simulink model "nxtmouse"  (Simulink 6.4)
settings: Solver=ode4  StartTime=0.0  StopTime=inf  FixedStep=Ts  RelTol=1e-3
PreLoadFcn:
  | param;
values from neighbouring files (symbols this model uses):
  CAMERA_POS = [100 100]    [param.m]
  Cm = 9.00e-6    (= 9e-06)    [param.m]
  Cw = 9.00e-4    (= 0.0009)    [param.m]
  Dx = 1e-3    (= 0.001)    [param.m]
  Dzz = 1e-6    (= 1e-06)    [param.m]
  e = -0.2    [param.m]
  J = M*(W/2)^2    (= 0.004096)    [param.m]
  Jm = 0.5e-7    (= 5e-08)    [param.m]
  Jw = 20.0e-7    (= 2e-06)    [param.m]
  Kb = 0.022    [param.m]
  Kt = 0.022    [param.m]
  LENGTH = 20    [param.m]
  LENGTH2 = 16    [param.m]
  Lm = 1.4e-3    (= 0.0014)    [param.m]
  M = 0.64    [param.m]
  n = 24    [param.m]
  Rm = 1.0    (= 1)    [param.m]
  Rw = 0.056/2    (= 0.028)    [param.m]
  START_POS = [22 15]    [param.m]
  TRACK_MAP = double(imread('track.bmp'))    [param.m]
  Ts = 0.0001    [param.m]
  W = 0.16    [param.m]
  WALL_MAP = ~(TRACK_MAP - WALL)    [param.m]
  WIDTH = 16    [param.m]
  WIDTH1 = 12    [param.m]
undefined symbols (not defined in the file or in its folder): clearNXTSignalObjects, DiscIntNeverNeededParam
libraries: simulink x13, vrlib x1, ecrobot_nxt_lib x1
(part 1 of 3)
settings Model: LastModifiedBy=takashic  ProdHWDeviceType=ARM7
settings DataIOCC: LimitDataPoints=off  SaveOutput=off  SignalLogging=off  SaveTime=off
settings OptimizationCC: InlineParams=on  InlineInvariantSignals=on  EnforceIntegerDowncast=off  StateBitsets=on  DataBitsets=on  UseTempVars=on  ZeroExternalMemoryAtStartup=off  ZeroInternalMemoryAtStartup=off  NoFixptDivByZeroProtection=on  EfficientFloat2IntCast=on  OptimizeModelRefInitCode=on  LifeSpan=1
settings DebuggingCC: ReadBeforeWriteMsg=DisableAll  WriteAfterWriteMsg=DisableAll  WriteAfterReadMsg=DisableAll  MultiTaskDSMMsg=none  ParameterDowncastMsg=warning  ParameterOverflowMsg=warning  ParameterUnderflowMsg=warning
settings HardwareCC: ProdIntDivRoundTo=Zero  ProdEndianess=LittleEndian  ProdHWDeviceType=ARM7
settings RTWCC: SystemTargetFile=ert.tlc  GenCodeOnly=on  TemplateMakefile=ert_default_tmf  Description=Real-Time Workshop Embedded Coder (no auto configuration)  RTWVerbose=off  ProcessScript=ert_make_rtw_hook
settings CodeAppCC: IgnoreCustomStorageClasses=off
settings ERTTargetCC: TargetFcnLib=ansi_tfl_tmw.mat  GenFloatMathFcnCalls=ANSI_C  IncludeMdlTerminateFcn=off  SuppressErrorStatus=on  IncludeERTFirstTime=on  SupportAbsoluteTime=off  SupportNonFinite=off  SupportComplex=off  InlinedParameterPlacement=NonHierarchical  ERTCustomFileTemplate=example_file_process.tlc  InitialValueSource=Model

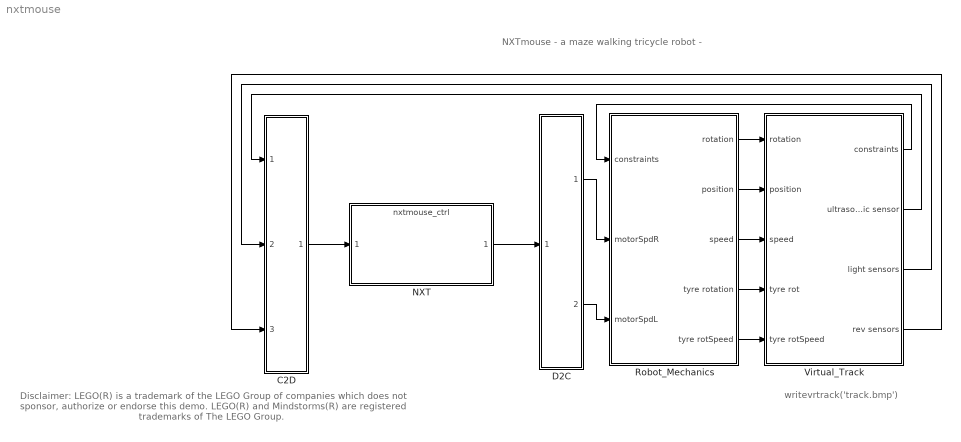
== system nxtmouse ==
  note: NXTmouse - a maze walking tricycle robot -
  note: writevrtrack('track.bmp')
  note: Disclaimer:
      | LEGO(R) is a trademark of the LEGO Group of companies which does not sponsor, authorize or endorse this demo.
      | LEGO(R) and Mindstorms(R)  are registered trademarks of The LEGO Group.
  C2D : Subsystem
  D2C : Subsystem
  NXT : ModelReference  StartFcn=%clearNXTSignalObjects();  ModelName=nxtmouse_ctrl  ModelReferenceVersion=1.499  CopyOfModelName=nxtmouse_ctrl
      mask init:
      | [data, map]=imread('NXT_ICON.gif');
      | pic=ind2rgb(data,map);
      mask Display: image(pic,  [45, 8, 50, 50])
  Robot_Mechanics : Subsystem
  Virtual_Track : Subsystem
  wires:
  Robot_Mechanics/2(position) -> Virtual_Track/2(position)
  Virtual_Track/1(constraints) -> Robot_Mechanics/1(constraints)
  Virtual_Track/3(light sensors) -> C2D/2(lights)
  C2D/1(Out1) -> NXT/1
  NXT/1 -> D2C/1(In1)
  D2C/2(motL) -> Robot_Mechanics/3(motorSpdL)
  Robot_Mechanics/1(rotation) -> Virtual_Track/1(rotation)
  D2C/1(motR) -> Robot_Mechanics/2(motorSpdR)
  Robot_Mechanics/4(tyre rotation) -> Virtual_Track/4(tyre rot)
  Robot_Mechanics/3(speed) -> Virtual_Track/3(speed)
  Robot_Mechanics/5(tyre rotSpeed) -> Virtual_Track/5(tyre rotSpeed)
  Virtual_Track/4(rev sensors) -> C2D/3(revs)
  Virtual_Track/2(ultrasonic sensor) -> C2D/1(sonar)

== system nxtmouse/C2D ==
  sonar : Inport
  lights : Inport  Port=2
  revs : Inport  Port=3
  Bus Creator : BusCreator  Inputs=5  UseBusObject=on
      settings: BusObject=Inputs
  Data Type Conversion1 : DataTypeConversion
  Data Type Conversion2 : DataTypeConversion
  Data Type Conversion5 : DataTypeConversion
  Demux1 : Demux  Outputs=2
  Demux2 : Demux  Outputs=2
  Zero-Order Hold1 : ZeroOrderHold  SampleTime=Ts*10
  Zero-Order Hold2 : ZeroOrderHold  SampleTime=Ts*10
  Zero-Order Hold3 : ZeroOrderHold  SampleTime=Ts*10
  Out1 : Outport
  wires:
  Zero-Order Hold2/1 -> Data Type Conversion2/1
  Zero-Order Hold1/1 -> Data Type Conversion1/1
  Data Type Conversion2/1 -> Demux1/1
  Bus Creator/1 -> Out1/1
  lights/1 -> Zero-Order Hold1/1
  revs/1 -> Zero-Order Hold2/1
  Zero-Order Hold3/1 -> Data Type Conversion5/1
  sonar/1 -> Zero-Order Hold3/1
  Data Type Conversion5/1 -> Bus Creator/1  "In_Sonar"
  Demux2/1 -> Bus Creator/2  "In_LightR"
  Demux2/2 -> Bus Creator/3  "In_LightL"
  Data Type Conversion1/1 -> Demux2/1
  Demux1/1 -> Bus Creator/4  "In_RevR"
  Demux1/2 -> Bus Creator/5  "In_RevL"

== system nxtmouse/D2C ==
  In1 : Inport
  Bus Selector : BusSelector  OutputSignals=Out_motorSpdR,Out_motorSpdL
  Data Type Conversion3 : DataTypeConversion  OutDataTypeMode=double
  Data Type Conversion5 : DataTypeConversion  OutDataTypeMode=double
  Rate Transition4 : RateTransition  Integrity=off  OutPortSampleTime=0
  Rate Transition6 : RateTransition  Integrity=off  OutPortSampleTime=0
  motR : Outport
  motL : Outport  Port=2
  wires:
  Bus Selector/1 -> Data Type Conversion3/1  "<Out_motorSpdR>"
  Bus Selector/2 -> Data Type Conversion5/1  "<Out_motorSpdL>"
  In1/1 -> Bus Selector/1
  Data Type Conversion3/1 -> Rate Transition4/1
  Data Type Conversion5/1 -> Rate Transition6/1
  Rate Transition4/1 -> motR/1
  Rate Transition6/1 -> motL/1

== system nxtmouse/Robot_Mechanics ==
  constraints : Inport
  motorSpdR : Inport  Port=2
  motorSpdL : Inport  Port=3
  Demux : Demux  Outputs=2
  Integrator2 : Integrator  UpperSaturationLimit=1e6  LowerSaturationLimit=-1e6
  Mux3 : Mux  Inputs=2
  Mux4 : Mux  Inputs=2
  Powertrain : Subsystem
  Product : Product  RndMeth=Zero
  Product1 : Product  RndMeth=Zero
  Saturation1 : Saturate  UpperLimit=1  LowerLimit=-1
  calc positoin[x z] : Subsystem
  percent2Ratio : Gain  Gain=1/100
  random gain : Subsystem
  random gain1 : Subsystem
  supplied voltage : Gain  Gain=8.25
  rotation : Outport
  position : Outport  Port=2
  speed : Outport  Port=3
  tyre rotation : Outport  Port=4
  tyre rotSpeed : Outport  Port=5
  wires:
  Demux/2 -> Powertrain/3(V_L)
  Demux/1 -> Powertrain/2(V_R)
  supplied voltage/1 -> Demux/1
  calc positoin[x z]/1(Out1) -> position/1
  constraints/1 -> Powertrain/1(constraints)
  Powertrain/3(RotV_R) -> Mux4/1
  Powertrain/4(RotV_L) -> Mux4/2
  Mux4/1 -> tyre rotSpeed/1, Integrator2/1
  Saturation1/1 -> supplied voltage/1
  Powertrain/2(Rotation) -> calc positoin[x z]/2(In2), rotation/1
  Powertrain/1(Forward_V) -> calc positoin[x z]/1(In1), speed/1
  Integrator2/1 -> tyre rotation/1
  percent2Ratio/1 -> Saturation1/1
  Mux3/1 -> percent2Ratio/1
  motorSpdR/1 -> Product/2
  Product/1 -> Mux3/1
  random gain/1(gain) -> Product/1
  Product1/1 -> Mux3/2
  motorSpdL/1 -> Product1/1
  random gain1/1(gain) -> Product1/2

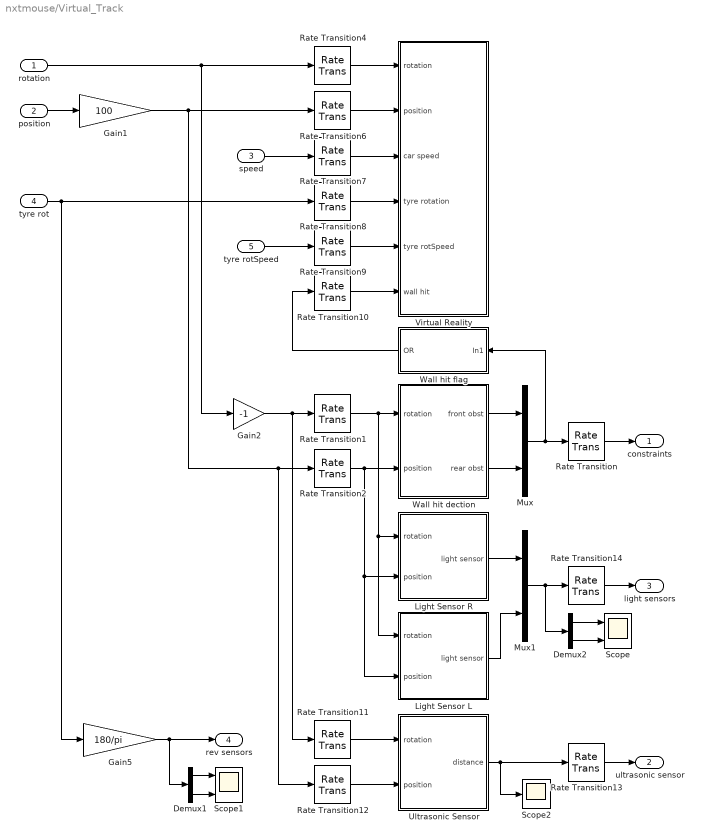
== system nxtmouse/Virtual_Track ==
  rotation : Inport
  position : Inport  Port=2
  speed : Inport  Port=3
  tyre rot : Inport  Port=4
  tyre rotSpeed : Inport  Port=5
  Demux1 : Demux  Outputs=2
  Demux2 : Demux  Outputs=2
  Gain1 : Gain  Gain=100
  Gain2 : Gain  Gain=-1
  Gain5 : Gain  Gain=180/pi
  Light Sensor L : Subsystem
  Light Sensor R : Subsystem
  Mux : Mux  Inputs=2
  Mux1 : Mux  Inputs=2
  Rate Transition : RateTransition  Integrity=off  OutPortSampleTime=0
  Rate Transition1 : RateTransition  Integrity=off  Deterministic=off  OutPortSampleTime=Ts*20
  Rate Transition{4,6..10} (6 alike) : RateTransition  Integrity=off  Deterministic=off  OutPortSampleTime=VR_TS
  Rate Transition11 : RateTransition  Integrity=off  Deterministic=off  OutPortSampleTime=Ts*500
  Rate Transition12 : RateTransition  Integrity=off  Deterministic=off  OutPortSampleTime=Ts*500
  Rate Transition13 : RateTransition  Integrity=off  Deterministic=off  OutPortSampleTime=Ts*10
  Rate Transition14 : RateTransition  Integrity=off  Deterministic=off  OutPortSampleTime=Ts*10
  Rate Transition2 : RateTransition  Integrity=off  Deterministic=off  OutPortSampleTime=Ts*20
  Scope : Scope  NumInputPorts=2
      settings: TimeRange=10  YMin=500~500  YMax=700~700  SaveName=ScopeData5
  Scope1 : Scope  NumInputPorts=2
      settings: YMin=0~0  YMax=15000~15000  SaveName=ScopeData4
  Scope2 : Scope
      settings: TimeRange=10  YMax=255  SaveName=ScopeData7
  Ultrasonic Sensor : Subsystem
  Virtual Reality : Subsystem
  Wall hit dection : Subsystem
  Wall hit flag : Subsystem  Orientation=left
  constraints : Outport
  ultrasonic sensor : Outport  Port=2
  light sensors : Outport  Port=3
  rev sensors : Outport  Port=4
  wires:
  rotation/1 -> Rate Transition4/1, Gain2/1
  position/1 -> Gain1/1
  Wall hit dection/1(front obst) -> Mux/1
  Wall hit dection/2(rear obst) -> Mux/2
  Mux/1 -> Rate Transition/1, Wall hit flag/1(In1)
  Rate Transition/1 -> constraints/1
  Rate Transition1/1 -> Wall hit dection/1(rotation), Light Sensor R/1(rotation), Light Sensor L/1(rotation)
  Rate Transition2/1 -> Wall hit dection/2(position), Light Sensor R/2(position), Light Sensor L/2(position)
  tyre rot/1 -> Rate Transition8/1, Gain5/1
  speed/1 -> Rate Transition7/1
  Rate Transition4/1 -> Virtual Reality/1(rotation)
  Rate Transition7/1 -> Virtual Reality/3(car speed)
  Rate Transition8/1 -> Virtual Reality/4(tyre rotation)
  Rate Transition6/1 -> Virtual Reality/2(position)
  Gain1/1 -> Rate Transition6/1, Rate Transition2/1, Rate Transition12/1
  tyre rotSpeed/1 -> Rate Transition9/1
  Rate Transition9/1 -> Virtual Reality/5(tyre rotSpeed)
  Rate Transition10/1 -> Virtual Reality/6(wall hit)
  Wall hit flag/1(OR) -> Rate Transition10/1
  Gain2/1 -> Rate Transition1/1, Rate Transition11/1
  Mux1/1 -> Rate Transition14/1, Demux2/1
  Gain5/1 -> rev sensors/1, Demux1/1
  Demux1/1 -> Scope1/1
  Demux1/2 -> Scope1/2
  Rate Transition12/1 -> Ultrasonic Sensor/2(position)
  Rate Transition11/1 -> Ultrasonic Sensor/1(rotation)
  Ultrasonic Sensor/1(distance) -> Rate Transition13/1, Scope2/1
  Rate Transition13/1 -> ultrasonic sensor/1
  Light Sensor R/1(light sensor) -> Mux1/1
  Light Sensor L/1(light sensor) -> Mux1/2
  Demux2/1 -> Scope/1
  Demux2/2 -> Scope/2
  Rate Transition14/1 -> light sensors/1

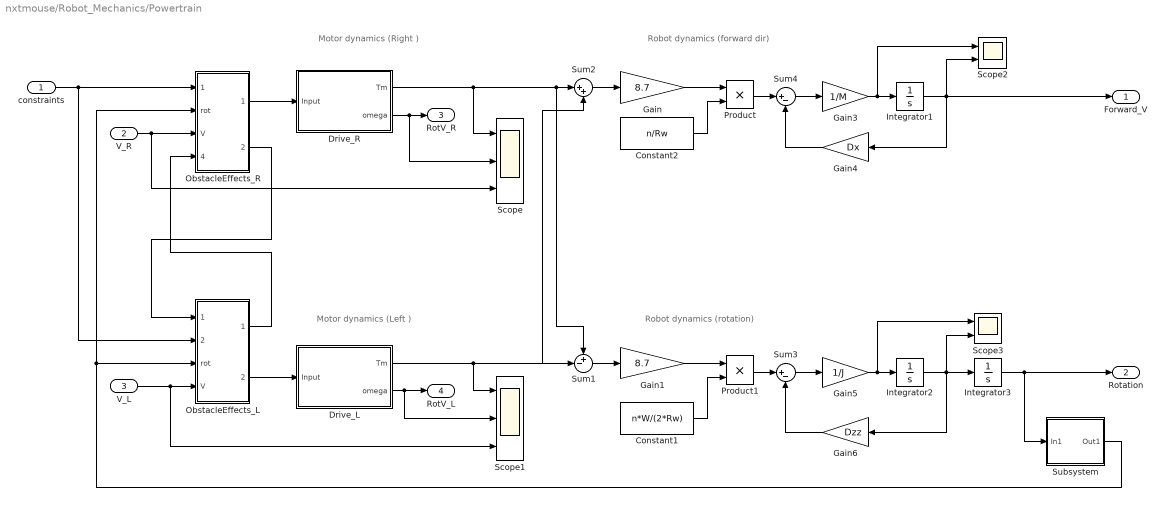
== system nxtmouse/Robot_Mechanics/Powertrain ==
  note: Motor dynamics (Right )
  note: Robot dynamics (forward dir)
  note: Motor dynamics (Left )
  note: Robot dynamics (rotation)
  constraints : Inport
  V_R : Inport  Port=2
  V_L : Inport  Port=3
  Constant1 : Constant  Value=n*W/(2*Rw)  OutDataType=sfix(16)  ConRadixGroup=Use specified scaling  OutScaling=2^0  SampleTime=inf  FramePeriod=inf
  Constant2 : Constant  Value=n/Rw  OutDataType=sfix(16)  ConRadixGroup=Use specified scaling  OutScaling=2^0  SampleTime=inf  FramePeriod=inf
  Drive_L : Subsystem
  Drive_R : Subsystem
  Gain : Gain  Gain=8.7
  Gain1 : Gain  Gain=8.7
  Gain3 : Gain  Gain=1/M
  Gain4 : Gain  Orientation=left  Gain=Dx
  Gain5 : Gain  Gain=1/J
  Gain6 : Gain  Orientation=left  Gain=Dzz
  Integrator1 : Integrator  UpperSaturationLimit=1e6  LowerSaturationLimit=-1e6
  Integrator2 : Integrator  UpperSaturationLimit=1e6  LowerSaturationLimit=-1e6
  Integrator3 : Integrator  UpperSaturationLimit=1e6  LowerSaturationLimit=-1e6
  ObstacleEffects_L : Subsystem
  ObstacleEffects_R : Subsystem
  Product : Product  RndMeth=Zero
  Product1 : Product  RndMeth=Zero
  Scope : Scope  NumInputPorts=3
      settings: TimeRange=9  YMin=-0.015~-100~-10  YMax=0.015~100~10
  Scope1 : Scope  NumInputPorts=3
      settings: TimeRange=10  YMin=-0.3~-15~-10  YMax=0.2~15~10
  Scope2 : Scope  NumInputPorts=2
      settings: TimeRange=3.5  YMin=-100~-1  YMax=200~2  SaveName=ScopeData2
  Scope3 : Scope  NumInputPorts=2
      settings: TimeRange=10  YMin=-2000~-10  YMax=2000~20  SaveName=ScopeData3
  Subsystem : Subsystem
  Sum1 : Sum  Inputs=+-|
  Sum2 : Sum  Inputs=|++
  Sum3 : Sum  Inputs=|+-
  Sum4 : Sum  Inputs=|+-
  Forward_V : Outport
  Rotation : Outport  Port=2
  RotV_R : Outport  Port=3
  RotV_L : Outport  Port=4
  wires:
  Drive_R/1(Tm) -> Scope/1, Sum2/1, Sum1/1
  Drive_L/1(Tm) -> Scope1/1, Sum1/2, Sum2/2
  Sum2/1 -> Gain/1
  Gain3/1 -> Scope2/1, Integrator1/1
  Integrator2/1 -> Scope3/2, Integrator3/1, Gain6/1
  Sum3/1 -> Gain5/1
  Constant2/1 -> Product/2
  Constant1/1 -> Product1/2
  Sum1/1 -> Gain1/1
  constraints/1 -> ObstacleEffects_R/1(constraints), ObstacleEffects_L/2(constraints)
  Gain6/1 -> Sum3/2
  Gain5/1 -> Integrator2/1, Scope3/1
  Product1/1 -> Sum3/1
  Sum4/1 -> Gain3/1
  Gain4/1 -> Sum4/2
  Product/1 -> Sum4/1
  V_R/1 -> Scope/3, ObstacleEffects_R/3(V)
  V_L/1 -> Scope1/3, ObstacleEffects_L/4(V)
  Drive_R/2(omega) -> RotV_R/1, Scope/2
  Drive_L/2(omega) -> RotV_L/1, Scope1/2
  ObstacleEffects_R/1(V_out) -> Drive_R/1(Input)
  ObstacleEffects_L/2(V_out) -> Drive_L/1(Input)
  Integrator1/1 -> Forward_V/1, Gain4/1, Scope2/2
  Integrator3/1 -> Rotation/1, Subsystem/1(In1)
  ObstacleEffects_L/1(restrct_R) -> ObstacleEffects_R/4(restrict)
  ObstacleEffects_R/2(restrict_L) -> ObstacleEffects_L/1(restrict)
  Gain/1 -> Product/1
  Gain1/1 -> Product1/1
  Subsystem/1(Out1) -> ObstacleEffects_L/3(rot), ObstacleEffects_R/2(rot)

== system nxtmouse/Robot_Mechanics/calc positoin[x z] ==
  In1 : Inport
  In2 : Inport  Port=2
  Integrator : Integrator
  Integrator1 : Integrator
  Mux1 : Mux  Inputs=2
  Product3 : Product  RndMeth=Zero
  Product4 : Product  RndMeth=Zero
  Trigonometric Function : Trigonometry  Operator=cos
  Trigonometric Function1 : Trigonometry
  Out1 : Outport
  wires:
  Integrator1/1 -> Mux1/2  "z"
  Product4/1 -> Integrator1/1
  Product3/1 -> Integrator/1
  Integrator/1 -> Mux1/1  "x"
  Trigonometric Function/1 -> Product3/1
  Trigonometric Function1/1 -> Product4/2
  In1/1 -> Product3/2, Product4/1
  Mux1/1 -> Out1/1
  In2/1 -> Trigonometric Function/1, Trigonometric Function1/1

== system nxtmouse/Robot_Mechanics/random gain ==
  Switch : Switch  Threshold=0.5
  sim While line1 : Constant  Value=rand  OutDataType=sfix(16)  ConRadixGroup=Use specified scaling  OutScaling=2^0  SampleTime=inf  FramePeriod=inf
  sim While line2 : Constant  Value=0.98  OutDataType=sfix(16)  ConRadixGroup=Use specified scaling  OutScaling=2^0  SampleTime=inf  FramePeriod=inf
  sim While line3 : Constant  Value=1  OutDataType=sfix(16)  ConRadixGroup=Use specified scaling  OutScaling=2^0  SampleTime=inf  FramePeriod=inf
  gain : Outport
  wires:
  sim While line1/1 -> Switch/2
  sim While line2/1 -> Switch/3
  sim While line3/1 -> Switch/1
  Switch/1 -> gain/1

== system nxtmouse/Robot_Mechanics/random gain1 ==
  Switch : Switch  Threshold=0.5
  sim While line1 : Constant  Value=rand  OutDataType=sfix(16)  ConRadixGroup=Use specified scaling  OutScaling=2^0  SampleTime=inf  FramePeriod=inf
  sim While line2 : Constant  Value=1  OutDataType=sfix(16)  ConRadixGroup=Use specified scaling  OutScaling=2^0  SampleTime=inf  FramePeriod=inf
  sim While line3 : Constant  Value=0.98  OutDataType=sfix(16)  ConRadixGroup=Use specified scaling  OutScaling=2^0  SampleTime=inf  FramePeriod=inf
  gain : Outport
  wires:
  Switch/1 -> gain/1
  sim While line3/1 -> Switch/1
  sim While line2/1 -> Switch/3
  sim While line1/1 -> Switch/2

== system nxtmouse/Virtual_Track/Light Sensor L ==
  rotation : Inport
  position : Inport  Port=2
  Fcn : Fcn  Expr=abs(rem(u[1], pi/2))
  Iterator : Stateflow chart
  Random Number : RandomNumber  Variance=0.1  SampleTime=Ts*20
  Ref : Subsystem
  Subsystem : Subsystem
  Sum : Sum  Inputs=|++
  light sensor : Outport
  wires:
  position/1 -> Subsystem/3(position)
  Iterator/1(range) -> Subsystem/1(range)
  Iterator/3(SearchObstacle) -> Subsystem/Trigger
  Subsystem/1(obst) -> Iterator/1(obstacle)
  Random Number/1 -> Iterator/2(noise)
  rotation/1 -> Fcn/1, Subsystem/2(rotation)
  Fcn/1 -> Iterator/3(rotation)
  Iterator/2(distance) -> Sum/1
  Sum/1 -> light sensor/1
  Ref/1(Out1) -> Sum/2

== system nxtmouse/Virtual_Track/Light Sensor R ==
  rotation : Inport
  position : Inport  Port=2
  Fcn : Fcn  Expr=abs(rem(u[1], pi/2))
  Iterator : Stateflow chart
  Random Number : RandomNumber  Variance=0.1  SampleTime=Ts*20
  Ref : Subsystem
  Subsystem : Subsystem
  Sum : Sum  Inputs=|++
  light sensor : Outport
  wires:
  Fcn/1 -> Iterator/3(rotation)
  rotation/1 -> Fcn/1, Subsystem/2(rotation)
  Random Number/1 -> Iterator/2(noise)
  Subsystem/1(obst) -> Iterator/1(obstacle)
  Iterator/1(range) -> Subsystem/1(range)
  position/1 -> Subsystem/3(position)
  Sum/1 -> light sensor/1
  Iterator/2(distance) -> Sum/1
  Ref/1(Out1) -> Sum/2
  Iterator/3(SearchObstacle) -> Subsystem/Trigger

== system nxtmouse/Virtual_Track/Ultrasonic Sensor ==
  rotation : Inport
  position : Inport  Port=2
  Constant : Constant  Value=LENGTH*0.5  OutDataType=sfix(16)  ConRadixGroup=Use specified scaling  OutScaling=2^0  SampleTime=inf  FramePeriod=inf
  Fcn : Fcn  Expr=abs(rem(u[1], pi/2))
  Iterator : Stateflow chart
  Random Number : RandomNumber  SampleTime=Ts*500
  Subsystem : Subsystem
  distance : Outport
  wires:
  position/1 -> Subsystem/3(position)
  Iterator/1(range) -> Subsystem/1(range)
  Iterator/3(SearchObstacle) -> Subsystem/Trigger
  Subsystem/1(front obst) -> Iterator/1(obstacle)
  Iterator/2(distance) -> distance/1
  Random Number/1 -> Iterator/3(noise)
  rotation/1 -> Subsystem/2(rotation), Fcn/1
  Fcn/1 -> Iterator/4(rotation)
  Constant/1 -> Iterator/2(offset)

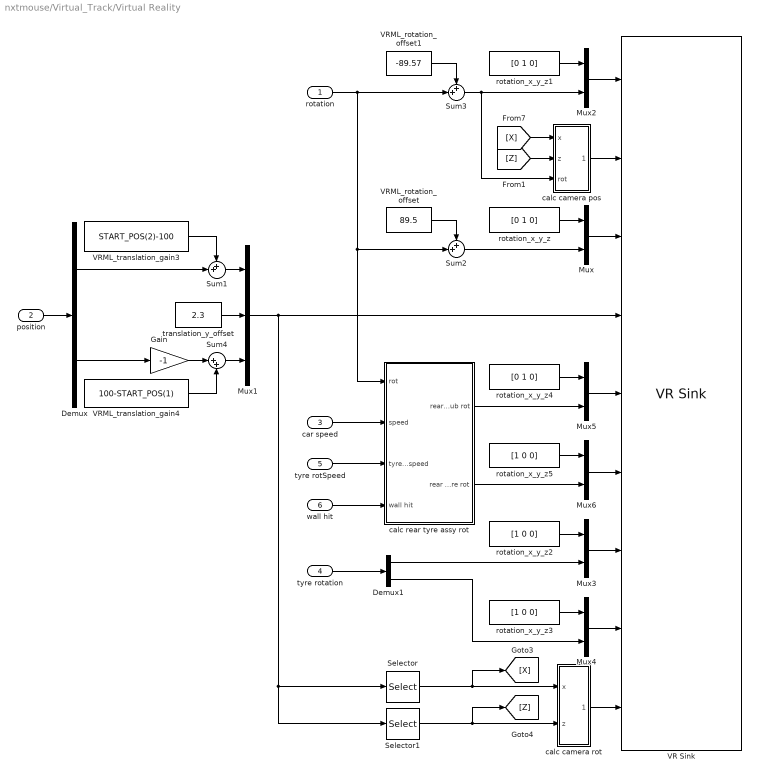
== system nxtmouse/Virtual_Track/Virtual Reality ==
  rotation : Inport
  position : Inport  Port=2
  car speed : Inport  Port=3
  tyre rotation : Inport  Port=4
  tyre rotSpeed : Inport  Port=5
  wall hit : Inport  Port=6
  " calc camera pos" : Subsystem
  Demux : Demux  Outputs=2
  Demux1 : Demux  Outputs=2
  Gain : Gain  Gain=-1
  Mux{,2..6} (6 alike) : Mux  Inputs=2
  Mux1 : Mux  Inputs=3
  Selector : Selector  InputPortWidth=3
  Selector1 : Selector  Elements=3  InputPortWidth=3
  Sum1 : Sum  Inputs=++|
  Sum2 : Sum  Inputs=++|
  Sum3 : Sum  Inputs=++|
  Sum4 : Sum  Inputs=|++
  VR Sink : vrlib/VR Sink  SampleTime=-1  ViewEnable=on  RemoteChange=off  RemoteView=off  FieldsWritten=OnBoardCamera.orientation.4.1.double#OnBoardCamera.position.3.1.double#NXT.rotation.4.1.double#NXT.translation.3.1.double#rearTyreAssy.rotation.4.1.double#Tyre.rotation.4.1.double#frontTyreR.rotation.4.1.double#frontTyreL.rotation.4.1.double#Camera.rotation.4.1.double  WorldFileName=vrnxtcartrack.wrl  AutoView=on  FigureProperties="{'Position', 'Name', 'Viewpoint', 'CameraBound', 'CameraDirection', 'CameraPosition', 'CameraUpVector', 'ZoomFactor', 'Antialiasing', 'Headlight', 'Lighting', 'NavPanel', 'StatusBar', 'ToolBar', 'Textures', 'Transparency', 'Wireframe', 'NavZones', 'NavMode', 'NavSpeed', 'Record2DCompressMethod', 'Record2DCompressQuality', 'Record2D', 'Record2DFileName'; [5.3800000000000000e+002  1.3100000000000000e+002  7.7300000000000000e+002  3.1800000000000000e+002], '', 'Chaser view', 'on', [0.0000000000000000e+000  0.0000000000000000e+000 -1.0000000000000000e+000], [0.0000000000000000e+000  0.0000000000000000e+000  0.0000000000000000e+000], [0.0000000000000000e+000  1.0000000000000000e+000  0.0000000000000000e+000], [1.0000000000000000e+000], 'on', 'off', 'on', 'none', 'on', 'on', 'on', 'on', 'off', 'off', 'walk', 'normal', 'auto', [7.5000000000000000e+001], 'off', '%f_anim_%n.avi'}"
  VRML_rotation_offset : Constant  Value=89.5  OutDataType=sfix(16)  ConRadixGroup=Use specified scaling  OutScaling=2^0  SampleTime=inf  FramePeriod=inf
  VRML_rotation_offset1 : Constant  Value=-89.57  OutDataType=sfix(16)  ConRadixGroup=Use specified scaling  OutScaling=2^0  SampleTime=inf  FramePeriod=inf
  VRML_translation_gain3 : Constant  Value=START_POS(2)-100  OutDataType=sfix(16)  ConRadixGroup=Use specified scaling  OutScaling=2^0  SampleTime=inf  FramePeriod=inf
  VRML_translation_gain4 : Constant  Value=100-START_POS(1)  OutDataType=sfix(16)  ConRadixGroup=Use specified scaling  OutScaling=2^0  SampleTime=inf  FramePeriod=inf
  calc camera rot : Subsystem
  calc rear tyre assy rot : Subsystem
  rotation_x_y_z : Constant  Value=[0 1 0]  OutDataType=sfix(16)  ConRadixGroup=Use specified scaling  OutScaling=2^0  SampleTime=inf  FramePeriod=inf
  rotation_x_y_z1 : Constant  Value=[0 1 0]  OutDataType=sfix(16)  ConRadixGroup=Use specified scaling  OutScaling=2^0  SampleTime=inf  FramePeriod=inf
  rotation_x_y_z2 : Constant  Value=[1 0 0]  OutDataType=sfix(16)  ConRadixGroup=Use specified scaling  OutScaling=2^0  SampleTime=inf  FramePeriod=inf
  rotation_x_y_z3 : Constant  Value=[1 0 0]  OutDataType=sfix(16)  ConRadixGroup=Use specified scaling  OutScaling=2^0  SampleTime=inf  FramePeriod=inf
  rotation_x_y_z4 : Constant  Value=[0 1 0]  OutDataType=sfix(16)  ConRadixGroup=Use specified scaling  OutScaling=2^0  SampleTime=inf  FramePeriod=inf
  rotation_x_y_z5 : Constant  Value=[1 0 0]  OutDataType=sfix(16)  ConRadixGroup=Use specified scaling  OutScaling=2^0  SampleTime=inf  FramePeriod=inf
  translation_y_offset : Constant  Value=2.3  OutDataType=sfix(16)  ConRadixGroup=Use specified scaling  OutScaling=2^0  SampleTime=inf  FramePeriod=inf
  wires:
  Selector/1 -> calc camera rot/1(x), [X]
  Selector1/1 -> calc camera rot/2(z), [Z]
  rotation/1 -> Sum3/2, Sum2/2, calc rear tyre assy rot/1(rot)
  VRML_rotation_offset/1 -> Sum2/1
  rotation_x_y_z/1 -> Mux/1
  Sum2/1 -> Mux/2
  Mux1/1 -> VR Sink/4, Selector1/1, Selector/1
  rotation_x_y_z1/1 -> Mux2/1
  Sum3/1 -> Mux2/2, " calc camera pos"/3(rot)
  VRML_rotation_offset1/1 -> Sum3/1
  [X] -> " calc camera pos"/1(x)
  translation_y_offset/1 -> Mux1/2
  Demux/1 -> Sum1/2
  position/1 -> Demux/1
  [Z] -> " calc camera pos"/2(z)
  Sum1/1 -> Mux1/1
  Sum4/1 -> Mux1/3
  Gain/1 -> Sum4/1
  VRML_translation_gain4/1 -> Sum4/2
  VRML_translation_gain3/1 -> Sum1/1
  Demux/2 -> Gain/1
  tyre rotation/1 -> Demux1/1
  rotation_x_y_z2/1 -> Mux3/1
  rotation_x_y_z3/1 -> Mux4/1
  Demux1/1 -> Mux3/2
  Demux1/2 -> Mux4/2
  rotation_x_y_z4/1 -> Mux5/1
  Mux2/1 -> VR Sink/1
  " calc camera pos"/1(Out1) -> VR Sink/2
  Mux/1 -> VR Sink/3
  Mux5/1 -> VR Sink/5
  Mux3/1 -> VR Sink/7
  Mux4/1 -> VR Sink/8
  Mux6/1 -> VR Sink/6
  rotation_x_y_z5/1 -> Mux6/1
  calc rear tyre assy rot/2(rear tyre rot) -> Mux6/2
  calc rear tyre assy rot/1(rear hub rot) -> Mux5/2
  tyre rotSpeed/1 -> calc rear tyre assy rot/3(tyre rot speed)
  wall hit/1 -> calc rear tyre assy rot/4(wall hit)
  car speed/1 -> calc rear tyre assy rot/2(speed)
  calc camera rot/1(rot) -> VR Sink/9

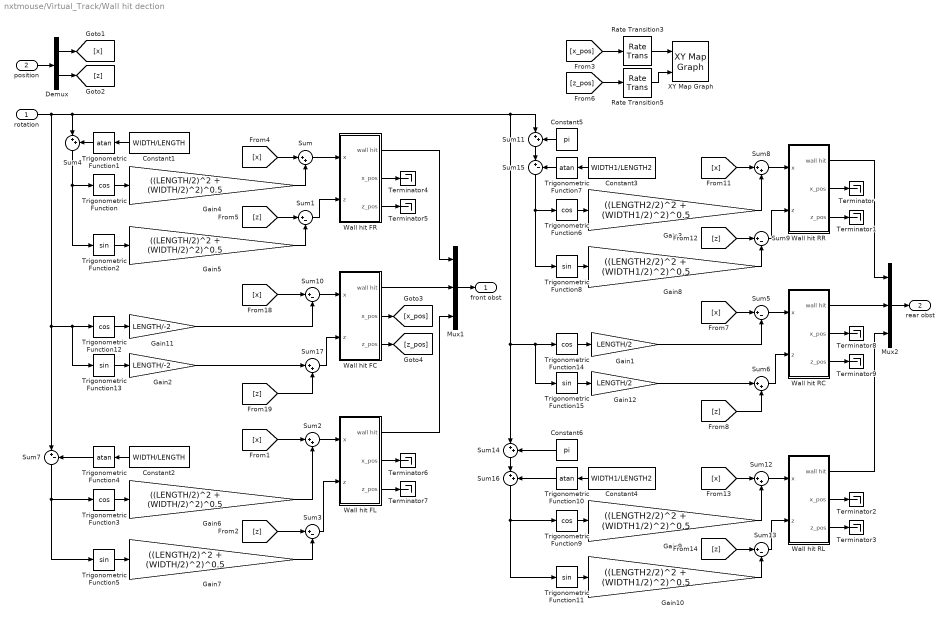
== system nxtmouse/Virtual_Track/Wall hit dection ==
  rotation : Inport
  position : Inport  Port=2
  Constant1 : Constant  Orientation=left  Value=WIDTH/LENGTH  OutDataType=sfix(16)  ConRadixGroup=Use specified scaling  OutScaling=2^0  SampleTime=inf  FramePeriod=inf
  Constant2 : Constant  Orientation=left  Value=WIDTH/LENGTH  OutDataType=sfix(16)  ConRadixGroup=Use specified scaling  OutScaling=2^0  SampleTime=inf  FramePeriod=inf
  Constant3 : Constant  Orientation=left  Value=WIDTH1/LENGTH2  OutDataType=sfix(16)  ConRadixGroup=Use specified scaling  OutScaling=2^0  SampleTime=inf  FramePeriod=inf
  Constant4 : Constant  Orientation=left  Value=WIDTH1/LENGTH2  OutDataType=sfix(16)  ConRadixGroup=Use specified scaling  OutScaling=2^0  SampleTime=inf  FramePeriod=inf
  Constant5 : Constant  Orientation=left  Value=pi  OutDataType=sfix(16)  ConRadixGroup=Use specified scaling  OutScaling=2^0  SampleTime=inf  FramePeriod=inf
  Constant6 : Constant  Orientation=left  Value=pi  OutDataType=sfix(16)  ConRadixGroup=Use specified scaling  OutScaling=2^0  SampleTime=inf  FramePeriod=inf
  Demux : Demux  Outputs=2
  Gain1 : Gain  Gain=LENGTH/2
  Gain{3,8..10} (4 alike) : Gain  Gain=((LENGTH2/2)^2 + (WIDTH1/2)^2)^0.5
  Gain11 : Gain  Gain=LENGTH/-2
  Gain12 : Gain  Gain=LENGTH/2
  Gain2 : Gain  Gain=LENGTH/-2
  Gain{4..7} (4 alike) : Gain  Gain=((LENGTH/2)^2 + (WIDTH/2)^2)^0.5
  Mux1 : Mux  Inputs=3
  Mux2 : Mux  Inputs=3
  Rate Transition3 : RateTransition  Integrity=off  Deterministic=off  OutPortSampleTime=Ts*1000
  Rate Transition5 : RateTransition  Integrity=off  Deterministic=off  OutPortSampleTime=Ts*1000
  Sum{,2,6,8,12,17} (6 alike) : Sum  Inputs=|++
  Sum{1,3,5,9..10,13} (6 alike) : Sum  Inputs=|+-
  Sum{4,11,14,16} (4 alike) : Sum  Orientation=down  Inputs=|++
  Sum15 : Sum  Orientation=down  Inputs=|+-
  Sum7 : Sum  Orientation=down  Inputs=|+-
  Terminator{,1..9} (10 alike) : Terminator
  Trigonometric Function{,3,6,9,12,14} (6 alike) : Trigonometry  Operator=cos
  Trigonometric Function{1,4,7,10} (4 alike) : Trigonometry  Orientation=left  Operator=atan
  Trigonometric Function{2,5,8,11,13,15} (6 alike) : Trigonometry
  Wall hit FC : Subsystem
  Wall hit FL : Subsystem
  Wall hit FR : Subsystem
  Wall hit RC : Subsystem
  Wall hit RL : Subsystem
  Wall hit RR : Subsystem
  XY Map Graph : ecrobot_nxt_lib/Utilities for simulation/XY Map Graph  SystemSampleTime=-1  xmin=0  xmax=200  ymin=0  ymax=200  map=TRACK_MAP
  front obst : Outport
  rear obst : Outport  Port=2
  wires:
  Gain9/1 -> Sum12/2
  Wall hit FC/3(z_pos) -> [z_pos]
  Wall hit RC/3(z_pos) -> Terminator9/1
  Wall hit RC/2(x_pos) -> Terminator8/1
  Mux2/1 -> rear obst/1
  Wall hit RL/1(wall hit) -> Mux2/3
  Wall hit RC/1(wall hit) -> Mux2/2
  Wall hit RR/1(wall hit) -> Mux2/1
  [z] -> Sum6/2
  [x] -> Sum5/1
  Sum5/1 -> Wall hit RC/1(x)
  Gain12/1 -> Sum6/1
  Sum6/1 -> Wall hit RC/2(z)
  Trigonometric Function14/1 -> Gain1/1
  Gain1/1 -> Sum5/2
  Trigonometric Function15/1 -> Gain12/1
  Wall hit FL/1(wall hit) -> Mux1/3
  [z] -> Sum17/2
  [x] -> Sum10/1
  Sum10/1 -> Wall hit FC/1(x)
  Gain2/1 -> Sum17/1
  Sum17/1 -> Wall hit FC/2(z)
  Trigonometric Function12/1 -> Gain11/1
  Gain11/1 -> Sum10/2
  Trigonometric Function13/1 -> Gain2/1
  Wall hit FC/1(wall hit) -> Mux1/2
  Wall hit FC/2(x_pos) -> [x_pos]
  position/1 -> Demux/1
  Wall hit RL/3(z_pos) -> Terminator3/1
  Wall hit RL/2(x_pos) -> Terminator2/1
  Wall hit RR/3(z_pos) -> Terminator1/1
  Wall hit RR/2(x_pos) -> Terminator/1
  Wall hit FR/3(z_pos) -> Terminator5/1
  Sum3/1 -> Wall hit FL/2(z)
  Trigonometric Function1/1 -> Sum4/2
  Constant1/1 -> Trigonometric Function1/1
  Wall hit FR/1(wall hit) -> Mux1/1
  Wall hit FR/2(x_pos) -> Terminator4/1
  Wall hit FL/2(x_pos) -> Terminator6/1
  Wall hit FL/3(z_pos) -> Terminator7/1
  Sum/1 -> Wall hit FR/1(x)
  [z] -> Sum1/1
  [x] -> Sum/1
  Trigonometric Function/1 -> Gain4/1
  Trigonometric Function2/1 -> Gain5/1
  Sum1/1 -> Wall hit FR/2(z)
  Sum4/1 -> Trigonometric Function2/1, Trigonometric Function/1
  Gain5/1 -> Sum1/2
  Gain4/1 -> Sum/2
  Sum2/1 -> Wall hit FL/1(x)
  [z] -> Sum3/1
  [x] -> Sum2/1
  Trigonometric Function3/1 -> Gain6/1
  Trigonometric Function5/1 -> Gain7/1
  Sum7/1 -> Trigonometric Function5/1, Trigonometric Function3/1
  Trigonometric Function4/1 -> Sum7/2
  Constant2/1 -> Trigonometric Function4/1
  Gain7/1 -> Sum3/2
  Gain6/1 -> Sum2/2
  [z] -> Sum9/1
  [x] -> Sum8/1
  Trigonometric Function6/1 -> Gain3/1
  Trigonometric Function8/1 -> Gain8/1
  Constant3/1 -> Trigonometric Function7/1
  Gain8/1 -> Sum9/2
  Gain3/1 -> Sum8/2
  Sum9/1 -> Wall hit RR/2(z)
  Sum8/1 -> Wall hit RR/1(x)
  [z] -> Sum13/1
  [x] -> Sum12/1
  Trigonometric Function9/1 -> Gain9/1
  Trigonometric Function11/1 -> Gain10/1
  Constant4/1 -> Trigonometric Function10/1
  Gain10/1 -> Sum13/2
  Sum12/1 -> Wall hit RL/1(x)
  Sum13/1 -> Wall hit RL/2(z)
  Sum11/1 -> Sum15/1
  Sum15/1 -> Trigonometric Function8/1, Trigonometric Function6/1
  Sum14/1 -> Sum16/1
  Sum16/1 -> Trigonometric Function11/1, Trigonometric Function9/1
  Trigonometric Function10/1 -> Sum16/2
  Constant6/1 -> Sum14/2
  Trigonometric Function7/1 -> Sum15/2
  Constant5/1 -> Sum11/2
  Mux1/1 -> front obst/1
  rotation/1 -> Sum4/1, Trigonometric Function14/1, Trigonometric Function15/1, Sum14/1, Sum11/1, Trigonometric Function13/1, Trigonometric Function12/1, Sum7/1
  Demux/2 -> [z]
  Demux/1 -> [x]
  Rate Transition3/1 -> XY Map Graph/1
  Rate Transition5/1 -> XY Map Graph/2
  [x_pos] -> Rate Transition3/1
  [z_pos] -> Rate Transition5/1

== system nxtmouse/Virtual_Track/Wall hit flag ==
  In1 : Inport
  Demux : Demux  Outputs=6
  Logical Operator : Logic  Operator=OR  Inputs=6  AllPortsSameDT=off  OutDataTypeMode=Boolean
  OR : Outport
  wires:
  In1/1 -> Demux/1
  Demux/1 -> Logical Operator/1
  Demux/2 -> Logical Operator/2
  Demux/3 -> Logical Operator/3
  Demux/4 -> Logical Operator/4
  Demux/5 -> Logical Operator/5
  Demux/6 -> Logical Operator/6
  Logical Operator/1 -> OR/1

== system nxtmouse/Robot_Mechanics/Powertrain/Drive_L ==
  Input : Inport
  Backlash : Backlash  BacklashWidth=bl
  Gain : Gain  Gain=1/Lm
  Gain1 : Gain  Orientation=left  Gain=Rm
  Gain10 : Gain  Orientation=left  Gain=Kb
  Gain11 : Gain  Orientation=left  Gain=Jm
  Gain2 : Gain  Gain=Kt
  Gain3 : Gain  Gain=1/Jm
  Gain4 : Gain  Orientation=left  Gain=Cw
  Gain5 : Gain  Orientation=left  Gain=1/n
  Gain6 : Gain  Orientation=left  Gain=1/n
  Gain7 : Gain  Orientation=left  Gain=Cm
  Gain8 : Gain  Gain=1/n
  Gain9 : Gain  Orientation=left  Gain=Jw
  Integrator : Integrator
  Integrator1 : Integrator
  Manual Switch : simulink/Signal Routing/Manual Switch  SystemSampleTime=-1  sw=0  action=0
  Step : Step  After=9  SampleTime=0
  Sum : Sum  Inputs=-+-
  Sum1 : Sum  Inputs=-+-
  Sum2 : Sum  Orientation=left  Inputs=|++
  Sum3 : Sum  Orientation=left  Inputs=|++
  Transfer Fcn : TransferFcn  Orientation=down  Numerator=[1 0]  Denominator=[0.1 1]
  Tm : Outport
  omega : Outport  Port=2
  wires:
  Backlash/1 -> Tm/1, Gain3/1
  Gain11/1 -> Sum2/1
  Gain5/1 -> Sum2/2  "Tw"
  Sum2/1 -> Sum1/3
  Step/1 -> Manual Switch/1
  Input/1 -> Manual Switch/2
  Manual Switch/1 -> Sum/2
  Gain8/1 -> Gain4/1, omega/1  "omega_w"
  Gain9/1 -> Sum3/1
  Gain4/1 -> Sum3/2  "Twv"
  Transfer Fcn/1 -> Gain11/1, Gain6/1
  Sum3/1 -> Gain5/1
  Gain6/1 -> Gain9/1
  Gain10/1 -> Sum/1  "Vb"
  Integrator1/1 -> Transfer Fcn/1, Gain8/1, Gain7/1, Gain10/1  "omega_m"
  Gain7/1 -> Sum1/1  "Tmv"
  Gain3/1 -> Integrator1/1
  Sum1/1 -> Backlash/1  "Tm"
  Gain2/1 -> Sum1/2  "T"
  Gain1/1 -> Sum/3  "Vr"
  Integrator/1 -> Gain1/1, Gain2/1  "i"
  Gain/1 -> Integrator/1
  Sum/1 -> Gain/1  "VLm"

== system nxtmouse/Robot_Mechanics/Powertrain/Drive_R ==
  Input : Inport
  Backlash : Backlash  BacklashWidth=bl
  Gain : Gain  Gain=1/Lm
  Gain1 : Gain  Orientation=left  Gain=Rm
  Gain10 : Gain  Orientation=left  Gain=Kb
  Gain11 : Gain  Orientation=left  Gain=Jm
  Gain2 : Gain  Gain=Kt
  Gain3 : Gain  Gain=1/Jm
  Gain4 : Gain  Orientation=left  Gain=Cw
  Gain5 : Gain  Orientation=left  Gain=1/n
  Gain6 : Gain  Orientation=left  Gain=1/n
  Gain7 : Gain  Orientation=left  Gain=Cm
  Gain8 : Gain  Gain=1/n
  Gain9 : Gain  Orientation=left  Gain=Jw
  Integrator : Integrator
  Integrator1 : Integrator
  Manual Switch : simulink/Signal Routing/Manual Switch  SystemSampleTime=-1  sw=0  action=0
  Step : Step  After=9  SampleTime=0
  Sum : Sum  Inputs=-+-
  Sum1 : Sum  Inputs=-+-
  Sum2 : Sum  Orientation=left  Inputs=|++
  Sum3 : Sum  Orientation=left  Inputs=|++
  Transfer Fcn : TransferFcn  Orientation=down  Numerator=[1 0]  Denominator=[0.1 1]
  Tm : Outport
  omega : Outport  Port=2
  wires:
  Sum/1 -> Gain/1  "VLm"
  Gain/1 -> Integrator/1
  Integrator/1 -> Gain2/1, Gain1/1  "i"
  Gain1/1 -> Sum/3  "Vr"
  Gain2/1 -> Sum1/2  "T"
  Sum1/1 -> Backlash/1  "Tm"
  Gain3/1 -> Integrator1/1
  Gain7/1 -> Sum1/1  "Tmv"
  Integrator1/1 -> Gain10/1, Gain7/1, Gain8/1, Transfer Fcn/1  "omega_m"
  Gain10/1 -> Sum/1  "Vb"
  Gain6/1 -> Gain9/1
  Sum3/1 -> Gain5/1
  Transfer Fcn/1 -> Gain6/1, Gain11/1
  Gain4/1 -> Sum3/2  "Twv"
  Gain9/1 -> Sum3/1
  Gain8/1 -> omega/1, Gain4/1  "omega_w"
  Manual Switch/1 -> Sum/2
  Input/1 -> Manual Switch/2
  Step/1 -> Manual Switch/1
  Sum2/1 -> Sum1/3
  Gain5/1 -> Sum2/2  "Tw"
  Gain11/1 -> Sum2/1
  Backlash/1 -> Gain3/1, Tm/1

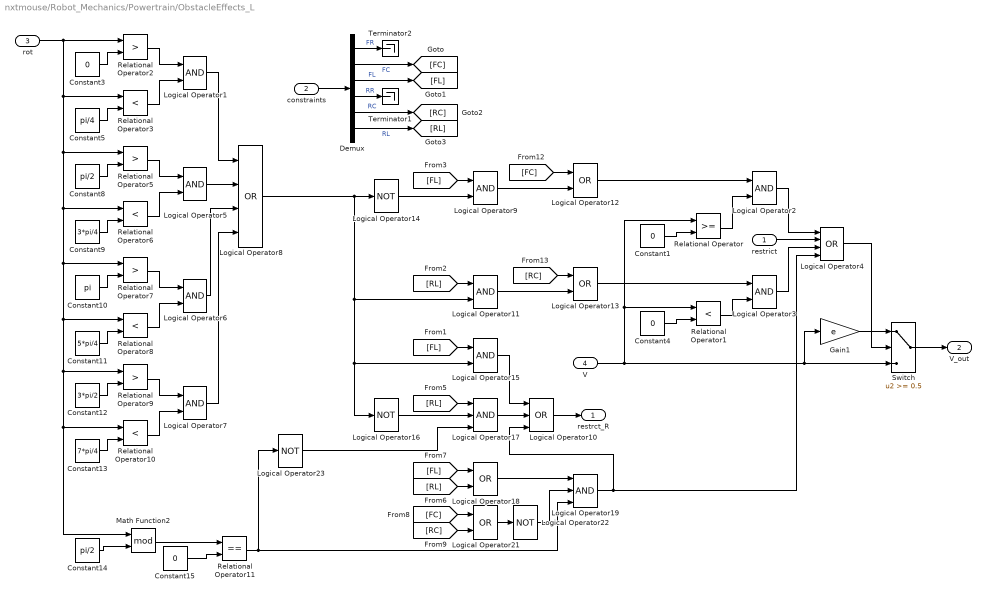
== system nxtmouse/Robot_Mechanics/Powertrain/ObstacleEffects_L ==
  restrict : Inport
  constraints : Inport  Port=2
  rot : Inport  Port=3
  V : Inport  Port=4
  Constant{1,3..4,15} (4 alike) : Constant  Value=0  OutDataType=sfix(16)  ConRadixGroup=Use specified scaling  OutScaling=2^0  SampleTime=inf  FramePeriod=inf
  Constant10 : Constant  Value=pi  OutDataType=sfix(16)  ConRadixGroup=Use specified scaling  OutScaling=2^0  SampleTime=inf  FramePeriod=inf
  Constant11 : Constant  Value=5*pi/4  OutDataType=sfix(16)  ConRadixGroup=Use specified scaling  OutScaling=2^0  SampleTime=inf  FramePeriod=inf
  Constant12 : Constant  Value=3*pi/2  OutDataType=sfix(16)  ConRadixGroup=Use specified scaling  OutScaling=2^0  SampleTime=inf  FramePeriod=inf
  Constant13 : Constant  Value=7*pi/4  OutDataType=sfix(16)  ConRadixGroup=Use specified scaling  OutScaling=2^0  SampleTime=inf  FramePeriod=inf
  Constant14 : Constant  Value=pi/2  OutDataType=sfix(16)  ConRadixGroup=Use specified scaling  OutScaling=2^0  SampleTime=inf  FramePeriod=inf
  Constant5 : Constant  Value=pi/4  OutDataType=sfix(16)  ConRadixGroup=Use specified scaling  OutScaling=2^0  SampleTime=inf  FramePeriod=inf
  Constant8 : Constant  Value=pi/2  OutDataType=sfix(16)  ConRadixGroup=Use specified scaling  OutScaling=2^0  SampleTime=inf  FramePeriod=inf
  Constant9 : Constant  Value=3*pi/4  OutDataType=sfix(16)  ConRadixGroup=Use specified scaling  OutScaling=2^0  SampleTime=inf  FramePeriod=inf
  Demux : Demux  Outputs=6
  Gain1 : Gain  Gain=e
  Logical Operator{1..3,5..7,9,11,15} (9 alike) : Logic  AllPortsSameDT=off  OutDataTypeMode=Boolean
  Logical Operator10 : Logic  Operator=OR  Inputs=3  AllPortsSameDT=off  OutDataTypeMode=Boolean
  Logical Operator{12..13,18,21} (4 alike) : Logic  Operator=OR  AllPortsSameDT=off  OutDataTypeMode=Boolean
  Logical Operator{14,16,22..23} (4 alike) : Logic  Operator=NOT  AllPortsSameDT=off  OutDataTypeMode=Boolean
  Logical Operator17 : Logic  Inputs=3  AllPortsSameDT=off  OutDataTypeMode=Boolean
  Logical Operator19 : Logic  Inputs=3  AllPortsSameDT=off  OutDataTypeMode=Boolean
  Logical Operator4 : Logic  Operator=OR  Inputs=4  AllPortsSameDT=off  OutDataTypeMode=Boolean
  Logical Operator8 : Logic  Operator=OR  Inputs=4  AllPortsSameDT=off  OutDataTypeMode=Boolean
  Math Function2 : Math  Operator=mod  SaturateOnIntegerOverflow=on
  Relational Operator : RelationalOperator  LogicOutDataTypeMode=Boolean
  Relational Operator{1,3,6,8,10} (5 alike) : RelationalOperator  Operator=<  LogicOutDataTypeMode=Boolean
  Relational Operator11 : RelationalOperator  Operator===  LogicOutDataTypeMode=Boolean
  Relational Operator{2,5,7,9} (4 alike) : RelationalOperator  Operator=>  LogicOutDataTypeMode=Boolean
  Switch : Switch  Threshold=0.5
  Terminator1 : Terminator
  Terminator2 : Terminator
  restrct_R : Outport
  V_out : Outport  Port=2
  wires:
  Logical Operator12/1 -> Logical Operator2/1
  [RC] -> Logical Operator13/1
  Logical Operator11/1 -> Logical Operator13/2
  [FC] -> Logical Operator12/1
  Logical Operator9/1 -> Logical Operator12/2
  [RL] -> Logical Operator11/1
  Logical Operator8/1 -> Logical Operator14/1, Logical Operator11/2, Logical Operator15/2, Logical Operator16/1
  Logical Operator7/1 -> Logical Operator8/4
  Logical Operator6/1 -> Logical Operator8/3
  Logical Operator5/1 -> Logical Operator8/2
  Logical Operator1/1 -> Logical Operator8/1
  Relational Operator10/1 -> Logical Operator7/2
  Relational Operator9/1 -> Logical Operator7/1
  Constant13/1 -> Relational Operator10/2
  Constant12/1 -> Relational Operator9/2
  Relational Operator8/1 -> Logical Operator6/2
  Relational Operator7/1 -> Logical Operator6/1
  Constant10/1 -> Relational Operator7/2
  Relational Operator6/1 -> Logical Operator5/2
  Relational Operator5/1 -> Logical Operator5/1
  Constant9/1 -> Relational Operator6/2
  Constant8/1 -> Relational Operator5/2
  rot/1 -> Relational Operator3/1, Relational Operator5/1, Relational Operator6/1, Relational Operator7/1, Relational Operator8/1, Relational Operator9/1, Relational Operator10/1, Math Function2/1, Relational Operator2/1
  Relational Operator3/1 -> Logical Operator1/2
  Relational Operator2/1 -> Logical Operator1/1
  Constant5/1 -> Relational Operator3/2
  Constant3/1 -> Relational Operator2/2
  Logical Operator4/1 -> Switch/2
  Logical Operator2/1 -> Logical Operator4/1
  Constant4/1 -> Relational Operator1/2
  Constant1/1 -> Relational Operator/2
  Relational Operator1/1 -> Logical Operator3/2
  Logical Operator13/1 -> Logical Operator3/1
  Relational Operator/1 -> Logical Operator2/2
  constraints/1 -> Demux/1
  Demux/1 -> Terminator2/1  "FR"
  Demux/4 -> Terminator1/1  "RR"
  Demux/2 -> [FC]  "FC"
  Demux/3 -> [FL]  "FL"
  Demux/5 -> [RC]  "RC"
  Demux/6 -> [RL]  "RL"
  Logical Operator14/1 -> Logical Operator9/2
  [FL] -> Logical Operator9/1
  Logical Operator10/1 -> restrct_R/1
  Logical Operator3/1 -> Logical Operator4/3
  restrict/1 -> Logical Operator4/2
  [FL] -> Logical Operator15/1
  [RL] -> Logical Operator17/1
  Logical Operator16/1 -> Logical Operator17/2
  Logical Operator15/1 -> Logical Operator10/1
  Logical Operator17/1 -> Logical Operator10/2
  Constant14/1 -> Math Function2/2
  [FL] -> Logical Operator18/1
  [RL] -> Logical Operator18/2
  Logical Operator18/1 -> Logical Operator19/1
  Logical Operator19/1 -> Logical Operator10/3, Logical Operator4/4
  [FC] -> Logical Operator21/1
  [RC] -> Logical Operator21/2
  Logical Operator21/1 -> Logical Operator22/1
  Relational Operator11/1 -> Logical Operator19/3, Logical Operator23/1
  Logical Operator22/1 -> Logical Operator19/2
  Gain1/1 -> Switch/1
  Constant11/1 -> Relational Operator8/2
  Constant15/1 -> Relational Operator11/2
  Math Function2/1 -> Relational Operator11/1
  Logical Operator23/1 -> Logical Operator17/3
  Switch/1 -> V_out/1
  V/1 -> Switch/3, Gain1/1, Relational Operator1/1, Relational Operator/1

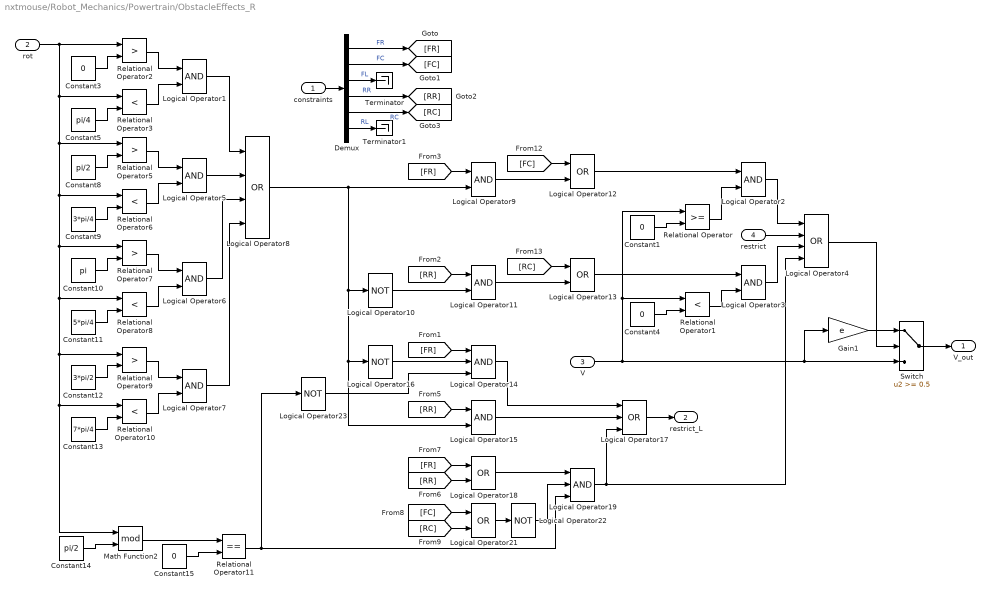
== system nxtmouse/Robot_Mechanics/Powertrain/ObstacleEffects_R ==
  constraints : Inport
  rot : Inport  Port=2
  V : Inport  Port=3
  restrict : Inport  Port=4
  Constant{1,3..4,15} (4 alike) : Constant  Value=0  OutDataType=sfix(16)  ConRadixGroup=Use specified scaling  OutScaling=2^0  SampleTime=inf  FramePeriod=inf
  Constant10 : Constant  Value=pi  OutDataType=sfix(16)  ConRadixGroup=Use specified scaling  OutScaling=2^0  SampleTime=inf  FramePeriod=inf
  Constant11 : Constant  Value=5*pi/4  OutDataType=sfix(16)  ConRadixGroup=Use specified scaling  OutScaling=2^0  SampleTime=inf  FramePeriod=inf
  Constant12 : Constant  Value=3*pi/2  OutDataType=sfix(16)  ConRadixGroup=Use specified scaling  OutScaling=2^0  SampleTime=inf  FramePeriod=inf
  Constant13 : Constant  Value=7*pi/4  OutDataType=sfix(16)  ConRadixGroup=Use specified scaling  OutScaling=2^0  SampleTime=inf  FramePeriod=inf
  Constant14 : Constant  Value=pi/2  OutDataType=sfix(16)  ConRadixGroup=Use specified scaling  OutScaling=2^0  SampleTime=inf  FramePeriod=inf
  Constant5 : Constant  Value=pi/4  OutDataType=sfix(16)  ConRadixGroup=Use specified scaling  OutScaling=2^0  SampleTime=inf  FramePeriod=inf
  Constant8 : Constant  Value=pi/2  OutDataType=sfix(16)  ConRadixGroup=Use specified scaling  OutScaling=2^0  SampleTime=inf  FramePeriod=inf
  Constant9 : Constant  Value=3*pi/4  OutDataType=sfix(16)  ConRadixGroup=Use specified scaling  OutScaling=2^0  SampleTime=inf  FramePeriod=inf
  Demux : Demux  Outputs=6
  Gain1 : Gain  Gain=e
  Logical Operator{1..3,5..7,9,11,15} (9 alike) : Logic  AllPortsSameDT=off  OutDataTypeMode=Boolean
  Logical Operator{10,16,22..23} (4 alike) : Logic  Operator=NOT  AllPortsSameDT=off  OutDataTypeMode=Boolean
  Logical Operator{12..13,18,21} (4 alike) : Logic  Operator=OR  AllPortsSameDT=off  OutDataTypeMode=Boolean
  Logical Operator14 : Logic  Inputs=3  AllPortsSameDT=off  OutDataTypeMode=Boolean
  Logical Operator17 : Logic  Operator=OR  Inputs=3  AllPortsSameDT=off  OutDataTypeMode=Boolean
  Logical Operator19 : Logic  Inputs=3  AllPortsSameDT=off  OutDataTypeMode=Boolean
  Logical Operator4 : Logic  Operator=OR  Inputs=4  AllPortsSameDT=off  OutDataTypeMode=Boolean
  Logical Operator8 : Logic  Operator=OR  Inputs=4  AllPortsSameDT=off  OutDataTypeMode=Boolean
  Math Function2 : Math  Operator=mod  SaturateOnIntegerOverflow=on
  Relational Operator : RelationalOperator  LogicOutDataTypeMode=Boolean
  Relational Operator{1,3,6,8,10} (5 alike) : RelationalOperator  Operator=<  LogicOutDataTypeMode=Boolean
  Relational Operator11 : RelationalOperator  Operator===  LogicOutDataTypeMode=Boolean
  Relational Operator{2,5,7,9} (4 alike) : RelationalOperator  Operator=>  LogicOutDataTypeMode=Boolean
  Switch : Switch  Threshold=0.5
  Terminator : Terminator
  Terminator1 : Terminator
  V_out : Outport
  restrict_L : Outport  Port=2
  wires:
  constraints/1 -> Demux/1
  Demux/1 -> [FR]  "FR"
  Demux/2 -> [FC]  "FC"
  Demux/3 -> Terminator/1  "FL"
  Demux/6 -> Terminator1/1  "RL"
  Demux/4 -> [RR]  "RR"
  Demux/5 -> [RC]  "RC"
  Relational Operator/1 -> Logical Operator2/2
  Logical Operator13/1 -> Logical Operator3/1
  Relational Operator1/1 -> Logical Operator3/2
  Constant1/1 -> Relational Operator/2
  Constant4/1 -> Relational Operator1/2
  Logical Operator4/1 -> Switch/2
  Constant3/1 -> Relational Operator2/2
  Constant5/1 -> Relational Operator3/2
  Relational Operator2/1 -> Logical Operator1/1
  Relational Operator3/1 -> Logical Operator1/2
  rot/1 -> Relational Operator9/1, Relational Operator10/1, Math Function2/1, Relational Operator8/1, Relational Operator7/1, Relational Operator6/1, Relational Operator5/1, Relational Operator3/1, Relational Operator2/1
  Constant8/1 -> Relational Operator5/2
  Constant9/1 -> Relational Operator6/2
  Relational Operator5/1 -> Logical Operator5/1
  Relational Operator6/1 -> Logical Operator5/2
  Constant10/1 -> Relational Operator7/2
  Constant11/1 -> Relational Operator8/2
  Relational Operator7/1 -> Logical Operator6/1
  Relational Operator8/1 -> Logical Operator6/2
  Constant12/1 -> Relational Operator9/2
  Constant13/1 -> Relational Operator10/2
  Relational Operator9/1 -> Logical Operator7/1
  Relational Operator10/1 -> Logical Operator7/2
  Logical Operator1/1 -> Logical Operator8/1
  Logical Operator5/1 -> Logical Operator8/2
  Logical Operator6/1 -> Logical Operator8/3
  Logical Operator7/1 -> Logical Operator8/4
  Logical Operator8/1 -> Logical Operator9/2, Logical Operator10/1, Logical Operator15/2, Logical Operator16/1
  [FR] -> Logical Operator9/1
  Logical Operator10/1 -> Logical Operator11/2
  [RR] -> Logical Operator11/1
  Logical Operator9/1 -> Logical Operator12/2
  [FC] -> Logical Operator12/1
  Logical Operator11/1 -> Logical Operator13/2
  [RC] -> Logical Operator13/1
  Logical Operator12/1 -> Logical Operator2/1
  Logical Operator3/1 -> Logical Operator4/3
  Logical Operator2/1 -> Logical Operator4/1
  restrict/1 -> Logical Operator4/2
  [FR] -> Logical Operator14/1
  [RR] -> Logical Operator15/1
  Logical Operator16/1 -> Logical Operator14/2
  Logical Operator14/1 -> Logical Operator17/1
  Logical Operator15/1 -> Logical Operator17/2
  Logical Operator17/1 -> restrict_L/1
  [FR] -> Logical Operator18/1
  [RR] -> Logical Operator18/2
  Logical Operator18/1 -> Logical Operator19/1
  Switch/1 -> V_out/1
  Logical Operator19/1 -> Logical Operator17/3, Logical Operator4/4
  [FC] -> Logical Operator21/1
  [RC] -> Logical Operator21/2
  Relational Operator11/1 -> Logical Operator19/3, Logical Operator23/1
  Logical Operator21/1 -> Logical Operator22/1
  Logical Operator22/1 -> Logical Operator19/2
  Gain1/1 -> Switch/1
  Math Function2/1 -> Relational Operator11/1
  Constant15/1 -> Relational Operator11/2
  Logical Operator23/1 -> Logical Operator14/3
  V/1 -> Relational Operator/1, Relational Operator1/1, Switch/3, Gain1/1
  Constant14/1 -> Math Function2/2

== system nxtmouse/Robot_Mechanics/Powertrain/Subsystem ==
  In1 : Inport
  Constant1 : Constant  Value=2*pi  OutDataType=sfix(16)  ConRadixGroup=Use specified scaling  OutScaling=2^0  SampleTime=inf  FramePeriod=inf
  Constant4 : Constant  Value=2*pi  OutDataType=sfix(16)  ConRadixGroup=Use specified scaling  OutScaling=2^0  SampleTime=inf  FramePeriod=inf
  Constant5 : Constant  Value=0  OutDataType=sfix(16)  ConRadixGroup=Use specified scaling  OutScaling=2^0  SampleTime=inf  FramePeriod=inf
  Math Function2 : Math  Operator=mod  SaturateOnIntegerOverflow=on
  Relational Operator12 : RelationalOperator  LogicOutDataTypeMode=Boolean
  Sum5 : Sum  Inputs=|++
  Switch2 : Switch  Threshold=0.5
  Out1 : Outport
  wires:
  Math Function2/1 -> Sum5/1, Relational Operator12/1, Switch2/1
  Constant5/1 -> Relational Operator12/2
  Relational Operator12/1 -> Switch2/2
  Sum5/1 -> Switch2/3
  Constant4/1 -> Math Function2/2
  In1/1 -> Math Function2/1
  Switch2/1 -> Out1/1
  Constant1/1 -> Sum5/2

== system nxtmouse/Virtual_Track/Light Sensor L/Ref ==
  Constant : Constant  Value=650  OutDataType=sfix(16)  ConRadixGroup=Use specified scaling  OutScaling=2^0  SampleTime=inf  FramePeriod=inf
  Constant1 : Constant  Value=rand  OutDataType=sfix(16)  ConRadixGroup=Use specified scaling  OutScaling=2^0  SampleTime=inf  FramePeriod=inf
  Constant2 : Constant  Value=550  OutDataType=sfix(16)  ConRadixGroup=Use specified scaling  OutScaling=2^0  SampleTime=inf  FramePeriod=inf
  Switch : Switch  Threshold=0.5
  Out1 : Outport
  wires:
  Constant1/1 -> Switch/2
  Switch/1 -> Out1/1
  Constant/1 -> Switch/1
  Constant2/1 -> Switch/3

== system nxtmouse/Virtual_Track/Light Sensor L/Subsystem ==
  range : Inport
  rotation : Inport  Port=2
  position : Inport  Port=3
  Function : TriggerPort  TriggerType=function-call
  Constant1 : Constant  Orientation=left  Value=0.5*LENGTH  OutDataType=sfix(16)  ConRadixGroup=Use specified scaling  OutScaling=2^0  SampleTime=inf  FramePeriod=inf
  Constant3 : Constant  Value=0.5*WIDTH  OutDataType=sfix(16)  ConRadixGroup=Use specified scaling  OutScaling=2^0  SampleTime=inf  FramePeriod=inf
  Demux : Demux  Outputs=2
  Fcn : Fcn  Expr=(((LENGTH/2)^2 + u[1]^2)^0.5)*u[2]
  Fcn1 : Fcn  Expr=(((LENGTH/2)^2 + u[1]^2)^0.5)*u[2]
  Mux : Mux  Inputs=2
  Mux2 : Mux  Inputs=2
  Product : Product  Orientation=left  Inputs=*/  RndMeth=Zero
  Sensing FR : Subsystem
  Sum : Sum  Inputs=|++
  Sum1 : Sum  Inputs=|+-
  Sum2 : Sum  Inputs=|++
  Sum4 : Sum  Orientation=down  Inputs=+-|
  Terminator4 : Terminator
  Terminator5 : Terminator
  Trigonometric Function : Trigonometry  Operator=cos
  Trigonometric Function1 : Trigonometry  Orientation=left  Operator=atan
  Trigonometric Function2 : Trigonometry
  obst : Outport  InitialOutput=0
  wires:
  Trigonometric Function2/1 -> Mux2/2
  Mux2/1 -> Fcn1/1
  Fcn/1 -> Sum/2
  Mux/1 -> Fcn/1
  position/1 -> Demux/1
  Demux/1 -> [x]
  Demux/2 -> [z]
  rotation/1 -> Sum4/1
  Fcn1/1 -> Sum1/2
  Sum4/1 -> Trigonometric Function/1, Trigonometric Function2/1
  Sum1/1 -> Sensing FR/2(z)
  Trigonometric Function/1 -> Mux/2
  [x] -> Sum/1
  [z] -> Sum1/1
  Sum/1 -> Sensing FR/1(x)
  Sensing FR/2(x_pos) -> Terminator4/1
  Sensing FR/1(wall hit) -> obst/1
  Product/1 -> Trigonometric Function1/1
  Trigonometric Function1/1 -> Sum4/2
  Sensing FR/3(z_pos) -> Terminator5/1
  Constant1/1 -> Product/2
  Sum2/1 -> Product/1, Mux2/1, Mux/1
  Constant3/1 -> Sum2/1
  range/1 -> Sum2/2

== system nxtmouse/Virtual_Track/Light Sensor R/Ref ==
  Constant : Constant  Value=650  OutDataType=sfix(16)  ConRadixGroup=Use specified scaling  OutScaling=2^0  SampleTime=inf  FramePeriod=inf
  Constant1 : Constant  Value=rand  OutDataType=sfix(16)  ConRadixGroup=Use specified scaling  OutScaling=2^0  SampleTime=inf  FramePeriod=inf
  Constant2 : Constant  Value=550  OutDataType=sfix(16)  ConRadixGroup=Use specified scaling  OutScaling=2^0  SampleTime=inf  FramePeriod=inf
  Switch : Switch  Threshold=0.5
  Out1 : Outport
  wires:
  Constant1/1 -> Switch/2
  Switch/1 -> Out1/1
  Constant/1 -> Switch/1
  Constant2/1 -> Switch/3
